simulink library "wnnsinks"  (R2021b)
settings: Solver=VariableStepAuto  StartTime=0.0  StopTime=10.0  RelTol=1e-3
settings Model: Creator=20214358  LastModifiedBy=20214358

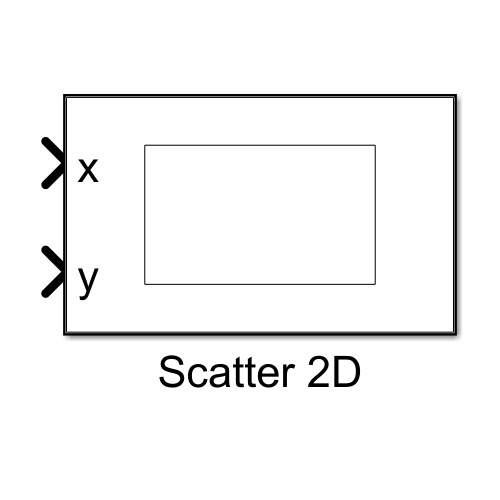
[thumbnail: Simulink's stored preview of the top-level diagram]
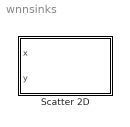
== system wnnsinks ==
  Scatter 2D : Subsystem
      mask Display:
      | port_label('input', 1,'x','interpreter','tex')
      | port_label('input', 2,'y','interpreter','tex')
      | pos = get_param(gcb, 'Position');
      | width = pos(3) - pos(1);
      | height = pos(4) - pos(2);
      | x = [0.2 0.8 0.8 0.2 0.2]*width;
      | y = [0.2 0.2 0.8 0.8 0.2]*height;
      | plot(x,y)
      | x = [0 1 1 0 0]*width;
      | y = [0 0 1 1 0]*height;
      | plot(x,y)

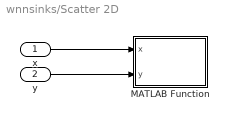
== system wnnsinks/Scatter 2D ==
  x : Inport
  y : Inport  Port=2
  MATLAB Function : MATLAB Function  TreatAsAtomicUnit=on
  wires:
  y/1 -> MATLAB Function/2(y)
  x/1 -> MATLAB Function/1(x)

== matlab function wnnsinks/Scatter 2D/MATLAB Function ==
  data: x input; y input
function fcn(x,y)

persistent hAxes

coder.extrinsic('scatter'); 

if isempty(hAxes)
    figure();
    hAxes = gca;
    hold on
end

scatter(hAxes,x,y)
